simulink model "model_T_PSH_IEEE39"  (R2020b)
settings: Solver=ode3  StartTime=0.0  StopTime=300  FixedStep=Ts  RelTol=1e-3
PostLoadFcn:
  | IEEE39BusLineLength;
  | vNomHV = 345E3;fNom=60;load('Dynamicload.mat');
InitFcn:
  | IEEE39BusLineLength;
  | vNomHV = 345E3;fNom=60;load('Dynamicload.mat');
values from neighbouring files (symbols this model uses):
  At = 1.48    [MAIN_T_PSH_IEEE39.m]
  Dturb = 0.3    [MAIN_T_PSH_IEEE39.m]
  fix_mode = 1    [MAIN_T_PSH_IEEE39.m]
  Gmax = 1    [MAIN_T_PSH_IEEE39.m]
  Gmin = 0    [MAIN_T_PSH_IEEE39.m]
  Hdam = 1    [MAIN_T_PSH_IEEE39.m]
  Kd = 1    [MAIN_T_PSH_IEEE39.m]    (also in plots_T_PSH_IEEE39.m)
  max_delay_gen2pump = 20    [MAIN_T_PSH_IEEE39.m]
  max_delay_pump2hsc = 30    [MAIN_T_PSH_IEEE39.m]
  pgen_pump = Kd*Pref    (= 0.9)    [MAIN_T_PSH_IEEE39.m]
  pgen_turb = (1-Kd)*Pref    (= 0)    [MAIN_T_PSH_IEEE39.m]
  pgen_turb_gen2pump = (1-kd_gen2pump)*Pref    (= 0)    [MAIN_T_PSH_IEEE39.m]
  pgen_turb_hsc2gen = (1-kd_hsc2gen)*Pref    (= 0.36)    [MAIN_T_PSH_IEEE39.m]
  pgen_turb_pump2hsc = (1-kd_pump2hsc)*Pref    (= 0.36)    [MAIN_T_PSH_IEEE39.m]
  Pref = 0.9    [MAIN_T_PSH_IEEE39.m]    (also in MAIN_VS_PSH.m = 1)
  qNL = 0.1    [MAIN_T_PSH_IEEE39.m]
  R = 0.04    [MAIN_T_PSH_IEEE39.m]
  r = 0.31    [MAIN_T_PSH_IEEE39.m]
  Rp = 0.05    [IEEE39BusLineLength.m]
  Sn = 320E6    (= 320000000)    [MAIN_T_PSH_IEEE39.m]
  t_gen2pump = 10    [MAIN_T_PSH_IEEE39.m]
  t_hsc2gen = 150    [MAIN_T_PSH_IEEE39.m]
  t_pump2hsc = 35    [MAIN_T_PSH_IEEE39.m]
  t_sw_off = 220    [MAIN_FS_PSH_IEEE39.m]    (also in MAIN_T_PSH_IEEE39.m; MAIN_VS_PSH.m = 45)
  t_sw_on = 130    [MAIN_FS_PSH_IEEE39.m]    (also in MAIN_T_PSH_IEEE39.m; MAIN_VS_PSH.m = 35)
  Tf = 0.05    [MAIN_T_PSH_IEEE39.m]
  Tg = 0.5    [MAIN_T_PSH_IEEE39.m]
  TL_10_11_len = 14    [IEEE39BusLineLength.m]
  TL_10_13_len = 14    [IEEE39BusLineLength.m]
  TL_13_14_len = 32    [IEEE39BusLineLength.m]
  TL_14_15_len = 70    [IEEE39BusLineLength.m]
  TL_15_16_len = 31.5    [IEEE39BusLineLength.m]
  TL_16_17_len = 26    [IEEE39BusLineLength.m]
  TL_16_19_len = 61    [IEEE39BusLineLength.m]
  TL_16_21_len = 46    [IEEE39BusLineLength.m]
  TL_16_24_len = 15    [IEEE39BusLineLength.m]
  TL_17_18_len = 26    [IEEE39BusLineLength.m]
  TL_17_27_len = 59    [IEEE39BusLineLength.m]
  TL_1_2_len = 134    [IEEE39BusLineLength.m]
  TL_1_39_len = 105    [IEEE39BusLineLength.m]
  TL_21_22_len = 47    [IEEE39BusLineLength.m]
  TL_22_23_len = 33    [IEEE39BusLineLength.m]
  TL_24_23_len = 88    [IEEE39BusLineLength.m]
  TL_25_26_len = 101    [IEEE39BusLineLength.m]
  TL_26_27_len = 46.5    [IEEE39BusLineLength.m]
  TL_26_28_len = 151    [IEEE39BusLineLength.m]
  TL_26_29_len = 200    [IEEE39BusLineLength.m]
  TL_28_29_len = 48    [IEEE39BusLineLength.m]
  TL_2_25_len = 28    [IEEE39BusLineLength.m]
  TL_2_2_len = 49    [IEEE39BusLineLength.m]
  TL_3_18_len = 42    [IEEE39BusLineLength.m]
  TL_3_4_len = 53    [IEEE39BusLineLength.m]
  TL_4_14_len = 33    [IEEE39BusLineLength.m]
  TL_4_5_len = 32.5    [IEEE39BusLineLength.m]
  TL_5_6_len = 14    [IEEE39BusLineLength.m]
  TL_5_8_len = 32    [IEEE39BusLineLength.m]
  TL_6_11_len = 26.5    [IEEE39BusLineLength.m]
  TL_6_7_len = 25.5    [IEEE39BusLineLength.m]
  TL_7_8_len = 15    [IEEE39BusLineLength.m]
  TL_8_9_len = 93    [IEEE39BusLineLength.m]
  TL_9_39_len = 136    [IEEE39BusLineLength.m]
  Tr = 6.88    [MAIN_T_PSH_IEEE39.m]
  Ts = 25e-6    (= 2.5e-05)    [MAIN_FS_PSH_IEEE39.m]    (also in MAIN_T_PSH_IEEE39.m; MAIN_VS_PSH.m = 1e-07)
  Velm = 0.05    [MAIN_T_PSH_IEEE39.m]
  Vn = 18000    [MAIN_T_PSH_IEEE39.m]
undefined symbols (not defined in the file or in its folder): D1, Delta, load15, load16, load18, load20, load21, load23, load24, load25, load26, load27, load28, load29, load3, load39, load4, load7, load8
libraries: powerlib x216, sps_avr x10, simulink_extras x7, powerlib_meascontrol x5, simulink x1
(part 1 of 9)
settings Model: ARTEMISmethode_block_infos=$$__separator__$$IEEE39bus_60Hz/ARTEMIS Guide$$__separator__$$  SimulationMode=accelerator  Creator=Admin  LastModifiedBy=mjimene
settings DataIOCC: LimitDataPoints=on  SaveFormat=Array  SignalLoggingSaveFormat=ModelDataLogs  SaveOutput=off  SignalLogging=off  DSMLogging=off  SaveTime=off
settings OptimizationCC: BlockReduction=off  OptimizeBlockIOStorage=off  BufferReuse=off  GlobalBufferReuse=off  ExpressionFolding=off  ExpressionDepthLimit=2147483647  LocalBlockOutputs=off  LifeSpan=inf
settings DebuggingCC: UnderspecifiedInitializationDetection=Classic  MergeDetectMultiDrivingBlocksExec=none  SolverPrmCheckMsg=warning  FcnCallInpInsideContextMsg=warning  UnconnectedInputMsg=none  UnconnectedOutputMsg=none  UnconnectedLineMsg=none  StateNameClashWarn=warning  SFUnexpectedBacktrackingDiag=warning  SFNoUnconditionalDefaultTransitionDiag=warning  SFExecutionAtInitializationDiag=none  ArithmeticOperatorsInVariantConditions=warning
settings HardwareCC: ProdBitPerPointer=32  ProdBitPerSizeT=32  ProdBitPerPtrDiffT=32  ProdLargestAtomicFloat=None  ProdIntDivRoundTo=Undefined  ProdEndianess=Unspecified  ProdWordSize=32  ProdHWDeviceType=32-bit Generic
settings ModelReferenceCC: PropagateSignalLabelsOutOfModel=off
settings SFSimCC: SimUseLocalCustomCode=off  CustomCodeUndefinedFunction=UseInterfaceOnly
settings RTWCC: RTWUseLocalCustomCode=off
settings CodeAppCC: StateflowObjectComments=on
settings GRTTargetCC: TargetLangStandard=C89/C90 (ANSI)  CombineOutputUpdateFcns=off  GRTInterface=on
settings ConfigComp: CovMetricSettings=dw  CovSaveCumulativeToWorkspaceVar=on  CovSaveSingleToWorkspaceVar=on  CovExternalEMLEnable=off
settings SimscapeCC: SimscapeNormalizeSystem=off

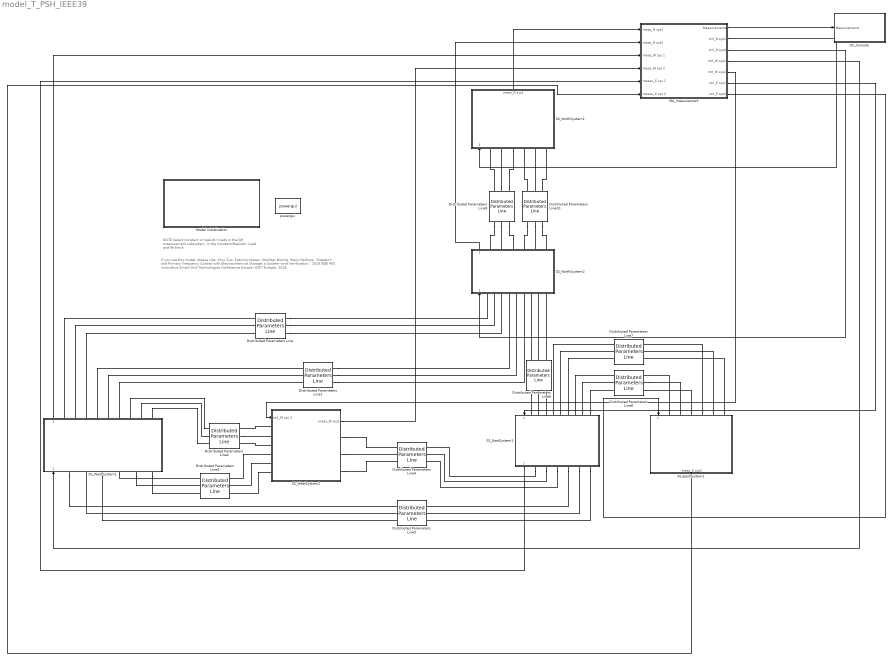
== system model_T_PSH_IEEE39 ==
  note: If you use this model, please cite:
      | Yihui Zuo, Fabrizio Sossan, Mokhtar Bozorg, Mario Paolone,
      | “Dispatch and Primary Frequency Control with Electrochemical Storage: a System-wise Verification,”
      | 2018 IEEE PES Innovative Smart Grid Technologies Conference Europe (ISGT-Europe), 2018.
  note: NOTE
      | Select constant or realistic loads in the SM measurement
      | subsystem, in the Constant/Realistic Load profile block.
  Distributed Parameters Line : powerlib/Elements/Distributed Parameters Line  Phases=3  Length=TL_1_39_len  Frequency=fNom  Resistance=[1.19 4.76]/TL_1_39_len  Inductance="[0.079  0.237]/TL_1_39_len"  Capacitance=[1.67e-6 0.7599e-6]/TL_1_39_len  x1=[-0.000425 6.82447359247909e-09 0 0;-0.0004 6.80872451608349e-09 0 0;-0.000375 6.79237064940765e-09 125916.274403475 -215667.287842067;-0.00035 6.77541344509656e-09 127943.255913456 -214470.993858132;-0.000325 6.75785440938716e-09 129958.872763666 -213255.64932043;-0.0003 6.73969510197452e-09 131962.945915361 -212021.362182889;-0.000275 6.72093713587333e-09 133955.297355178 -210768.242082031;-0.00025 6.7015821772746e-09 135935.75011094 -209496.400327228;-0.000225 6.68163194539767e-09 137904.128267383 -208205.949890819;-0.0002 6.66108821233747e-09 139860.256981778 -206897.005398072;-0.000175 6.63995280290718e-09 141803.962499462 -205569.683117007;-0.00015 6.61822759447605e-09 143735.072169272 -204224.100948063;-0.000125 6.59591451680273e-09 145653.414458882 -202860.378413628;-0.0001 6.57301555186379e-09 147558.818970036 -201478.636647424;-7.5e-05 6.5495327336777e-09 149451.116453689 -200078.998383743;-5e-05 6.52546814812414e-09 151330.138825038 -198661.587946549;-2.5e-05 6.50082393275876e-09 153195.719178451 -197226.531238432]  x2=[-0.000425 -1.36577479152877e-10 0 0;-0.0004 -1.69010241030866e-10 0 0;-0.000375 -2.01427990442011e-10 135245.30623613 -213822.142207347;-0.00035 -2.33827847854369e-10 137254.483681511 -212538.007509997;-0.000325 -2.66206935325264e-10 139251.469390032 -211234.993957904;-0.0003 -2.98562376756929e-10 141236.085977876 -209913.217292266;-0.000275 -3.30891298151972e-10 143208.157159922 -208572.794920929;-0.00025 -3.63190827868667e-10 145167.507765405 -207213.845907958;-0.000225 -3.95458096876025e-10 147113.963753475 -205836.490963062;-0.0002 -4.27690239008639e-10 149047.352228657 -204440.852430872;-0.000175 -4.59884391221277e-10 150967.501456207 -203027.054280071;-0.00015 -4.92037693843189e-10 152874.240877369 -201595.222092386;-0.000125 -5.24147290832123e-10 154767.401124522 -200145.483051432;-0.0001 -5.56210330028012e-10 156646.814036226 -198677.965931411;-7.5e-05 -5.88223963406325e-10 158512.31267216 -197192.80108568;-5e-05 -6.20185347331038e-10 160363.731327948 -195690.120435168;-2.5e-05 -6.52091642807227e-10 162200.90554988 -194170.05745666]  x3=[-0.000425 2.81520374156516e-11 0 0;-0.0004 2.73917536840612e-11 0 0;-0.000375 2.66290368585268e-11 583.079334168895 -1337.51010433723;-0.00035 2.58639546879668e-11 595.658933399881 -1331.95538957714;-0.000325 2.50965751314035e-11 608.185622760243 -1326.28236283785;-0.0003 2.4326966351926e-11 620.658289557001 -1320.49152803039;-0.000275 2.35551967106363e-11 633.075825895772 -1314.58339953019;-0.00025 2.27813347605761e-11 645.437128779179 -1308.5585021314;-0.000225 2.20054492406386e-11 657.741100204826 -1302.41737100023;-0.0002 2.12276090694618e-11 669.986647262827 -1296.16055162746;-0.000175 2.04478833393073e-11 682.172682232888 -1289.78859977996;-0.00015 1.96663413099229e-11 694.298122680923 -1283.30208145135;-0.000125 1.88830524023906e-11 706.361891555199 -1276.70157281168;-0.0001 1.80980861929602e-11 718.362917282012 -1269.98766015629;-7.5e-05 1.73115124068691e-11 730.300133860866 -1263.16093985374;-5e-05 1.65234009121492e-11 742.172480959161 -1256.22201829278;-2.5e-05 1.57338217134204e-11 753.978904006382 -1249.17151182855]  x4=[-0.000425 -1.66454786224224e-11 0 0;-0.0004 -1.59649069897711e-11 0 0;-0.000375 -1.52829172617703e-11 477.711890398408 -711.188785738365;-0.00035 -1.4599570016691e-11 484.393311485576 -706.654944302658;-0.000325 -1.39149259533866e-11 491.031705958008 -702.058333688848;-0.0003 -1.32290458859015e-11 497.626484155121 -697.399362194468;-0.000275 -1.25419907380692e-11 504.177060290586 -692.678443656305;-0.00025 -1.18538215381005e-11 510.682852504353 -687.89599741364;-0.000225 -1.11645994131627e-11 517.143282914341 -683.052448271001;-0.0002 -1.04743855839503e-11 523.557777667766 -678.148226460429;-0.000175 -9.78324135924631e-12 529.925766992116 -673.183767603262;-0.00015 -9.09122813047713e-12 536.246685245757 -668.15951267144;-0.000125 -8.39840736625901e-12 542.519970968182 -663.075907948337;-0.0001 -7.70484060693819e-12 548.745066929881 -657.933404989118;-7.5e-05 -7.01058945912449e-12 554.921420181837 -652.732460580631;-5e-05 -6.31571559021911e-12 561.04848210464 -647.473536700831;-2.5e-05 -5.62028072293689e-12 567.125708457224 -642.157100477745]  x5=0.000424377544174995  V1=ones(3,3)  V2=ones(3,3)  I1=ones(3,3)  I2=ones(3,3)  nHarmo=1  Measurements=None  Decoupling=off  VsMag0=0  VrMag0=0  VsAngle0=0  VrAngle0=0  IsMag0=0  IrMag0=0  IsAngle0=0  IrAngle0=0
  Distributed Parameters Line1 : powerlib/Elements/Distributed Parameters Line  Phases=3  Length=TL_3_4_len  Frequency=fNom  Resistance=[1.547 6.18]/TL_3_4_len  Inductance="[0.067  0.208]/TL_3_4_len"  Capacitance=[0.493e-6 0.224e-6]/TL_3_4_len  x1=[-0.000225 1.6958252968873e-09 0 0;-0.0002 1.54824975012124e-09 116464.900989505 -210886.461836935;-0.000175 1.40053667886024e-09 118447.246041312 -209779.455322648;-0.00015 1.25269920383338e-09 120419.069923853 -208653.814984172;-0.000125 1.10475045682001e-09 122380.197488327 -207509.640807393;-0.0001 9.56703579483276e-10 124330.454536047 -206347.034424475;-7.5e-05 8.08571722202861e-10 126269.667833903 -205166.09910484;-5e-05 6.60368042906836e-10 128197.665129758 -203966.939745992;-2.5e-05 5.12105705902926e-10 130114.275167745 -202749.662864199]  x2=[-0.000225 2.13834554662331e-09 0 0;-0.0002 2.00645197588943e-09 134479.442824576 -206334.576910516;-0.000175 1.87438018048954e-09 136418.087730126 -205057.992053123;-0.00015 1.74214189180416e-09 138344.61519234 -203763.19275921;-0.000125 1.60974885600272e-09 140258.85408591 -202450.294040337;-0.0001 1.47721283300015e-09 142160.634377069 -201119.412515759;-7.5e-05 1.34454559541237e-09 144049.787138696 -199770.666402069;-5e-05 1.21175892751051e-09 145926.14456532 -198404.175502695;-2.5e-05 1.07886462417419e-09 147789.539988023 -197020.06119726]  x3=[-0.000225 -1.78483661113028e-11 0 0;-0.0002 -1.79240452695748e-11 518.089821308726 -1279.69932908716;-0.000175 -1.79981323105074e-11 530.127485951711 -1274.75969133324;-0.00015 -1.80706206532611e-11 542.118061606143 -1269.70682205274;-0.000125 -1.81415038590023e-11 554.060483199762 -1264.54117007074;-0.0001 -1.82107756314747e-11 565.953689937629 -1259.2631942303;-7.5e-05 -1.8278429817559e-11 577.796625396356 -1253.87336335177;-5e-05 -1.83444604078192e-11 589.588237617937 -1248.37215619108;-2.5e-05 -1.84088615370365e-11 601.327479203194 -1242.76006139727]  x4=[-0.000225 2.50482695965397e-11 0 0;-0.0002 2.48471590066135e-11 121.777473885469 128.221815017289;-0.000175 2.46438413483556e-11 120.563589621472 129.363838061733;-0.00015 2.4438334681616e-11 119.338996202334 130.494370262086;-0.000125 2.42306572606851e-11 118.103802403524 131.61331119794;-0.0001 2.40208275326721e-11 116.858117942096 132.720561478492;-7.5e-05 2.38088641358669e-11 115.602053466947 133.81602275137;-5e-05 2.35947858980839e-11 114.335720548986 134.89959771137;-2.5e-05 2.337861183499e-11 113.059231671226 135.971190109098]  x5=0.000215851801011713  V1=ones(3,3)  V2=ones(3,3)  I1=ones(3,3)  I2=ones(3,3)  nHarmo=1  Measurements=None  Decoupling=off  VsMag0=0  VrMag0=0  VsAngle0=0  VrAngle0=0  IsMag0=0  IrMag0=0  IsAngle0=0  IrAngle0=0
  Distributed Parameters Line10 : powerlib/Elements/Distributed Parameters Line  Phases=3  Length=TL_2_25_len  Frequency=fNom  Resistance=[8.33 33.3]/TL_2_25_len  Inductance=[0.027 0.082]/TL_2_25_len  Capacitance=[0.325e-6 0.148e-6]/TL_2_25_len  x1=[-0.000125 -9.05757141638467e-09 0 0;-0.0001 -9.06957005980283e-09 167648.596320969 -188428.534351372;-7.5e-05 -9.08076309156712e-09 169417.00966394 -186840.137060953;-5e-05 -9.09114951744772e-09 171170.374408526 -185235.143549232;-2.5e-05 -9.10072841486225e-09 172908.534810733 -183613.696381013]  x2=[-0.000125 -4.26747363705766e-10 0 0;-0.0001 -6.61699299596901e-10 171332.219594936 -182512.291487725;-7.5e-05 -8.96592459530234e-10 173044.711024908 -180889.440362705;-5e-05 -1.13140597893712e-09 174741.831623084 -179250.521591671;-2.5e-05 -1.36611900032306e-09 176423.4306414 -177595.680752865]  x3=[-0.000125 4.70773669429525e-10 0 0;-0.0001 4.68396340500153e-10 1075.86934502619 -582.792909139489;-7.5e-05 4.65977405899503e-10 1081.31415478568 -572.627345310123;-5e-05 4.63517080491332e-10 1086.66291596967 -562.410917408958;-2.5e-05 4.61015582815971e-10 1091.91515347028 -552.144532918193]  x4=[-0.000125 -4.78403021988109e-10 0 0;-0.0001 -4.7636898850949e-10 52.6144484395538 -697.070225634231;-7.5e-05 -4.74292641182898e-10 59.181687592818 -696.543389127242;-5e-05 -4.72174164441509e-10 65.7436698863957 -695.954681608947;-2.5e-05 -4.70013746460675e-10 72.2998124470777 -695.304155371752]  x5=0.000110163514831363  V1=ones(3,3)  V2=ones(3,3)  I1=ones(3,3)  I2=ones(3,3)  nHarmo=1  Measurements=None  Decoupling=off  VsMag0=0  VrMag0=0  VsAngle0=0  VrAngle0=0  IsMag0=0  IrMag0=0  IsAngle0=0  IrAngle0=0
  Distributed Parameters Line2 : powerlib/Elements/Distributed Parameters Line  Phases=3  Length=TL_5_6_len  Frequency=fNom  Resistance=[0.476 1.904]/TL_5_6_len  Inductance=[0.014 0.04]/TL_5_6_len  Capacitance=[0.162e-6 0.074e-6]/TL_5_6_len  x1=[-7.5e-05 6.48469401785956e-09 0 0;-5e-05 6.33185153631539e-09 132982.125706271 -200175.622617078;-2.5e-05 6.17844662310637e-09 134862.791231139 -198913.421899552]  x2=[-7.5e-05 6.42421610984077e-09 0 0;-5e-05 6.25757145564951e-09 138041.32215589 -196698.021310076;-2.5e-05 6.09037096777966e-09 139888.987836916 -195388.293819903]  x3=[-7.5e-05 1.00931057100308e-10 0 0;-5e-05 1.00601283191749e-10 1184.48127250464 -1575.38524962129;-2.5e-05 1.00262573295529e-10 1199.27604059468 -1564.15196917421]  x4=[-7.5e-05 -8.68602062268655e-11 0 0;-5e-05 -8.69239264867509e-11 -275.774523608809 218.716848838573;-2.5e-05 -8.69799256608829e-11 -277.823617259088 216.10806706858]  x5=5.44058820349418e-05  V1=ones(3,3)  V2=ones(3,3)  I1=ones(3,3)  I2=ones(3,3)  nHarmo=1  Measurements=None  Decoupling=off  VsMag0=0  VrMag0=0  VsAngle0=0  VrAngle0=0  IsMag0=0  IrMag0=0  IsAngle0=0  IrAngle0=0
  Distributed Parameters Line3 : powerlib/Elements/Distributed Parameters Line  Phases=3  Length=TL_7_8_len  Frequency=fNom  Resistance=[0.476 1.904]/TL_7_8_len  Inductance=[0.015 0.044]/TL_7_8_len  Capacitance=[0.174e-6 0.079e-6]/TL_7_8_len  x1=[-7.5e-05 6.07040960241395e-09 122557.52009298 -206550.592006867;-5e-05 5.91980751784004e-09 124498.730220582 -205386.356365422;-2.5e-05 5.76867960173348e-09 126428.881651101 -204203.877120241]  x2=[-7.5e-05 6.76218751498753e-09 124786.001456704 -204826.24564208;-5e-05 6.61873636774516e-09 126710.861311159 -203641.083921901;-2.5e-05 6.47469730606841e-09 128624.465974257 -202437.833623176]  x3=[-7.5e-05 -3.90124045178195e-11 745.609660166508 -1072.1989685999;-5e-05 -3.88230244083392e-11 755.681589498115 -1065.12423419214;-2.5e-05 -3.86301958133523e-11 765.686394821515 -1057.95488929125]  x4=[-7.5e-05 4.65349128222633e-11 82.3065432237965 -335.30367631357;-5e-05 4.58823976117957e-11 85.4629698146192 -334.513076858687;-2.5e-05 4.52258068614755e-11 88.6118050903075 -333.692764018129]  x5=5.89576118919347e-05  V1=ones(3,3)  V2=ones(3,3)  I1=ones(3,3)  I2=ones(3,3)  nHarmo=1  Measurements=None  Decoupling=off  VsMag0=0  VrMag0=0  VsAngle0=0  VrAngle0=0  IsMag0=0  IrMag0=0  IsAngle0=0  IrAngle0=0
  Distributed Parameters Line4 : powerlib/Elements/Distributed Parameters Line  Phases=3  Length=TL_13_14_len  Frequency=fNom  Resistance=[1.071 4.285]/TL_13_14_len  Inductance=[0.032 0.095]/TL_13_14_len  Capacitance=[0.384e-6 0.175e-6]/TL_13_14_len  x1=[-0.00015 -1.84588646488538e-08 0 0;-0.000125 -1.85855470778483e-08 137054.160835711 -198017.584467246;-0.0001 -1.87105786310878e-08 138914.30756397 -196717.103644566;-7.5e-05 -1.88339482025469e-08 140762.115120216 -195399.149271302;-5e-05 -1.89556448338268e-08 142597.419371495 -194063.838415782;-2.5e-05 -1.90756577151292e-08 144420.057295474 -192711.289688038]  x2=[-0.00015 -1.82342608230128e-12 0 0;-0.000125 -1.73806690637535e-10 128270.609996984 -204367.02656213;-0.0001 -3.45774516677539e-10 130190.987834372 -203149.045137268;-7.5e-05 -5.17711629025669e-10 132099.801355444 -201913.018839589;-5e-05 -6.89602755233448e-10 133996.881008345 -200659.057460094;-2.5e-05 -8.61432626937154e-10 135882.058283491 -199387.272382886]  x3=[-0.00015 1.65856168110498e-10 0 0;-0.000125 1.70279111060999e-10 -126.262148596948 -18.9493361137516;-0.0001 1.74686928836284e-10 -126.078020265121 -20.1384817636324;-7.5e-05 1.79079229908492e-10 -125.882692954539 -21.3258385971202;-5e-05 1.83455624128046e-10 -125.676184015303 -22.5113011463157;-2.5e-05 1.87815722758306e-10 -125.458511790729 -23.6947641115808]  x4=[-0.00015 -1.89775651879871e-10 0 0;-0.000125 -1.94616313616103e-10 1013.74461396554 -1390.25070636974;-0.0001 -1.99439688406069e-10 1026.802198003 -1380.63477026534;-7.5e-05 -2.0424534780973e-10 1039.76857553216 -1370.89619819767;-5e-05 -2.09032864960632e-10 1052.6425948044 -1361.03585520302;-2.5e-05 -2.13801814603819e-10 1065.42311227488 -1351.05461713407]  x5=0.000128937969582276  V1=ones(3,3)  V2=ones(3,3)  I1=ones(3,3)  I2=ones(3,3)  nHarmo=1  Measurements=None  Decoupling=off  VsMag0=0  VrMag0=0  VsAngle0=0  VrAngle0=0  IsMag0=0  IrMag0=0  IsAngle0=0  IrAngle0=0
  Distributed Parameters Line5 : powerlib/Elements/Distributed Parameters Line  Phases=3  Length=TL_4_14_len  Frequency=fNom  Resistance=[0.9522 3.808]/TL_4_14_len  Inductance=[0.041 0.1223]/TL_4_14_len  Capacitance=[0.308e-6 0.14e-6]/TL_4_14_len  x1=[-0.00015 1.25269920383338e-09 0 0;-0.000125 1.10475045682001e-09 122380.197488327 -207509.640807393;-0.0001 9.56703579483276e-10 124330.454536047 -206347.034424475;-7.5e-05 8.08571722202861e-10 126269.667833903 -205166.09910484;-5e-05 6.60368042906836e-10 128197.665129758 -203966.939745992;-2.5e-05 5.12105705902926e-10 130114.275167745 -202749.662864199]  x2=[-0.00015 -1.82342608230128e-12 0 0;-0.000125 -1.73806690637535e-10 128270.609996984 -204367.02656213;-0.0001 -3.45774516677539e-10 130190.987834372 -203149.045137268;-7.5e-05 -5.17711629025669e-10 132099.801355444 -201913.018839589;-5e-05 -6.89602755233448e-10 133996.881008345 -200659.057460094;-2.5e-05 -8.61432626937154e-10 135882.058283491 -199387.272382886]  x3=[-0.00015 5.29965279778984e-11 0 0;-0.000125 5.25426459549767e-11 548.434518132287 -941.542402513085;-0.0001 5.20840967904346e-11 557.283853983036 -936.331761920028;-7.5e-05 5.162092121526e-11 566.083688659603 -931.037950925913;-5e-05 5.11531603713857e-11 574.83324050979 -925.661439757641;-2.5e-05 5.06808558080345e-11 583.531732347811 -920.202705988024]  x4=[-0.00015 -5.31610401189671e-11 0 0;-0.000125 -5.30486831737016e-11 113.330971162931 -199.672553983299;-0.0001 -5.29316141376637e-11 115.207723378569 -198.595605403815;-7.5e-05 -5.28098434096022e-11 117.074242178074 -197.50101641436;-5e-05 -5.26833818058973e-11 118.930361766454 -196.388884242657;-2.5e-05 -5.25522405595997e-11 120.775917272435 -195.259307674714]  x5=0.000130851060370178  V1=ones(3,3)  V2=ones(3,3)  I1=ones(3,3)  I2=ones(3,3)  nHarmo=1  Measurements=None  Decoupling=off  VsMag0=0  VrMag0=0  VsAngle0=0  VrAngle0=0  IsMag0=0  IrMag0=0  IsAngle0=0  IrAngle0=0
  Distributed Parameters Line6 : powerlib/Elements/Distributed Parameters Line  Phases=3  Length=TL_16_17_len  Frequency=fNom  Resistance=[0.8332 3.33]/TL_16_17_len  Inductance=[0.028 0.084]/TL_16_17_len  Capacitance=[0.299e-6 0.136e-6]/TL_16_17_len  x1=[-0.000125 3.55201829698564e-08 0 0;-0.0001 3.52355613436191e-08 127482.761229804 -209764.944408129;-7.5e-05 3.49478098910877e-08 129454.048045797 -208554.148041724;-5e-05 3.465695417201e-08 131413.836004727 -207324.826690009;-2.5e-05 3.43630200218728e-08 133361.951026895 -206077.089548415]  x2=[-0.000125 2.39408399520577e-08 0 0;-0.0001 2.36824783705596e-08 131020.122877065 -208712.127601341;-7.5e-05 2.34220131743981e-08 132981.329601984 -207468.039590694;-5e-05 2.31594674995981e-08 134930.724156296 -206205.523069169;-2.5e-05 2.28948646669843e-08 136868.133383506 -204924.690180784]  x3=[-0.000125 -7.51676539007504e-11 0 0;-0.0001 -7.88220241180392e-11 529.194411884565 -1016.0874974886;-7.5e-05 -8.24693929073891e-11 538.747124460212 -1011.05495400868;-5e-05 -8.61094362884146e-11 548.251982401175 -1005.93260278172;-2.5e-05 -8.97418309314155e-11 557.708141431012 -1000.72089880458]  x4=[-0.000125 1.53319636933556e-10 0 0;-0.0001 1.56315144972869e-10 290.26469102285 -363.176651707524;-7.5e-05 1.59296768197176e-10 293.674582186092 -360.424825714346;-5e-05 1.62264241761462e-10 297.058387474888 -357.640984704135;-2.5e-05 1.65217302077566e-10 300.415806320087 -354.825375953746]  x5=0.000106883113727099  V1=ones(3,3)  V2=ones(3,3)  I1=ones(3,3)  I2=ones(3,3)  nHarmo=1  Measurements=None  Decoupling=off  VsMag0=0  VrMag0=0  VsAngle0=0  VrAngle0=0  IsMag0=0  IrMag0=0  IsAngle0=0  IrAngle0=0
  Distributed Parameters Line7 : powerlib/Elements/Distributed Parameters Line  Phases=3  Length=TL_16_21_len  Frequency=fNom  Resistance=[0.9522 3.809]/TL_16_21_len  Inductance=[0.043 0.128]/TL_16_21_len  Capacitance=[0.568e-6 0.258e-6]/TL_16_21_len  x1=[-0.0002 3.63550174769137e-08 0 0;-0.000175 3.60799358967494e-08 121501.663663936 -213285.116380796;-0.00015 3.5801649488061e-08 123506.392436839 -212130.533640322;-0.000125 3.55201829698564e-08 125500.150657839 -210957.10823929;-0.0001 3.52355613436191e-08 127482.761229804 -209764.944408129;-7.5e-05 3.49478098910877e-08 129454.048045797 -208554.148041724;-5e-05 3.465695417201e-08 131413.836004727 -207324.826690009;-2.5e-05 3.43630200218728e-08 133361.951026895 -206077.089548415]  x2=[-0.0002 1.49365973206953e-08 0 0;-0.000175 1.46837342890637e-08 127042.880582269 -205846.70751626;-0.00015 1.44295669632497e-08 128977.258914018 -204640.23140741;-0.000125 1.41741179198648e-08 130900.180739872 -203415.577969956;-0.0001 1.39174098493701e-08 132811.475254794 -202172.855984697;-7.5e-05 1.36594655540607e-08 134710.972686554 -200912.175837386;-5e-05 1.34003079460404e-08 136598.504310808 -199633.649508922;-2.5e-05 1.31399600451864e-08 138473.902466083 -198337.390565408]  x3=[-0.0002 -2.79115737680193e-11 0 0;-0.000175 -3.24004215604224e-11 894.375330557269 -1099.60469305758;-0.00015 -3.68863913600399e-11 904.698963155013 -1091.12669262415;-0.000125 -4.13690846970961e-11 914.942235159789 -1082.55177200889;-0.0001 -4.58481033928492e-11 925.10423670495 -1073.88069288581;-7.5e-05 -5.03230495949607e-11 935.184065142762 -1065.1142254703;-5e-05 -5.47935258128342e-11 945.180825124579 -1056.25314845069;-2.5e-05 -5.92591349529233e-11 955.093628680379 -1047.29824891907]  x4=[-0.0002 1.03978847655996e-10 0 0;-0.000175 1.07755027360876e-10 -38.2016559913804 -446.336261559181;-0.00015 1.11521635641174e-10 -33.993452625192 -446.676471583733;-0.000125 1.15278337924966e-10 -29.7822297639879 -446.977005221351;-0.0001 1.19024800520232e-10 -25.5683614729324 -447.237835776899;-7.5e-05 1.22760690644503e-10 -21.352222052172 -447.4589400819;-5e-05 1.26485676454416e-10 -17.1341860035882 -447.64029849659;-2.5e-05 1.30199427075194e-10 -12.914627997532 -447.781894911666]  x5=0.000181725067065609  V1=ones(3,3)  V2=ones(3,3)  I1=ones(3,3)  I2=ones(3,3)  nHarmo=1  Measurements=None  Decoupling=off  VsMag0=0  VrMag0=0  VsAngle0=0  VrAngle0=0  IsMag0=0  IrMag0=0  IsAngle0=0  IrAngle0=0
  Distributed Parameters Line8 : powerlib/Elements/Distributed Parameters Line  Phases=3  Length=TL_16_24_len  Frequency=fNom  Resistance=[0.357 1.428]/TL_16_24_len  Inductance=[0.019 0.056]/TL_16_24_len  Capacitance=[0.152e-6 0.069e-6]/TL_16_24_len  x1=[-7.5e-05 3.49478098910877e-08 129454.048045797 -208554.148041724;-5e-05 3.465695417201e-08 131413.836004727 -207324.826690009;-2.5e-05 3.43630200218728e-08 133361.951026895 -206077.089548415]  x2=[-7.5e-05 2.9424529652556e-08 129729.694883358 -210501.804918846;-5e-05 2.91892483982628e-08 131707.826547799 -209269.799286697;-2.5e-05 2.89513743861516e-08 133674.259161538 -208019.205100957]  x3=[-7.5e-05 -2.51469137348881e-10 90.694597336161 -645.022035350488;-5e-05 -2.54078013566083e-10 96.7696531139891 -644.138623589418;-2.5e-05 -2.56664321105016e-10 102.836113251696 -643.197995711326]  x4=[-7.5e-05 3.22554721209669e-10 629.831976985986 -546.772388466727;-5e-05 3.24525319269697e-10 634.957095144396 -540.81216044826;-2.5e-05 3.26467091114429e-10 640.025812742229 -534.803894366671]  x5=6.21610810716802e-05  V1=ones(3,3)  V2=ones(3,3)  I1=ones(3,3)  I2=ones(3,3)  nHarmo=1  Measurements=None  Decoupling=off  VsMag0=0  VrMag0=0  VsAngle0=0  VrAngle0=0  IsMag0=0  IrMag0=0  IsAngle0=0  IrAngle0=0
  Distributed Parameters Line9 : powerlib/Elements/Distributed Parameters Line  Phases=3  Length=TL_26_27_len  Frequency=fNom  Resistance=[1.666 6.665]/TL_26_27_len  Inductance=[0.046 0.139]/TL_26_27_len  Capacitance=[0.534e-6 0.243e-6]/TL_26_27_len  x1=[-0.0002 1.52272838880291e-08 0 0;-0.000175 1.49472449786049e-08 127256.586831929 -211796.164829682;-0.00015 1.46658783684552e-08 129247.026043211 -210587.410058936;-0.000125 1.43832090501892e-08 131225.984786321 -209359.949696791;-0.0001 1.40992621321302e-08 133193.287278701 -208113.892773374;-7.5e-05 1.38140628360853e-08 135148.758773167 -206849.349970666;-5e-05 1.3527636495105e-08 137092.225573436 -205566.433612669;-2.5e-05 1.3240008551233e-08 139023.515049548 -204265.257655433]  x2=[-0.0002 9.02877067542436e-09 0 0;-0.000175 8.71213522248572e-09 141750.530907737 -204239.085171132;-0.00015 8.39472590732218e-09 143669.103226295 -202894.065812053;-0.000125 8.07657092406441e-09 145574.914024395 -201531.024228895;-0.0001 7.75769853307762e-09 147467.794016903 -200150.081494893;-7.5e-05 7.43813705845132e-09 149347.575067272 -198751.360273364;-5e-05 7.11791488548344e-09 151214.090202481 -197334.984806816;-2.5e-05 6.79706045815894e-09 153067.173627864 -195901.080905906]  x3=[-0.0002 8.02462137756003e-11 0 0;-0.000175 7.87138233867969e-11 920.624462147512 -1516.26187198719;-0.00015 7.71744411810691e-11 934.873751756558 -1507.51799994247;-0.000125 7.56282038952452e-11 949.040000473439 -1498.64022143237;-0.0001 7.40752488750614e-11 963.121949970034 -1489.62932503252;-7.5e-05 7.25157140629621e-11 977.118349406165 -1480.48611114283;-5e-05 7.09497379858465e-11 991.027955540705 -1471.21139191643;-2.5e-05 6.93774597427646e-11 1004.84953284201 -1461.80599118751]  x4=[-0.0002 -4.44685173545744e-11 0 0;-0.000175 -4.36928200540542e-11 -49.7397106711078 77.7795104983289;-0.00015 -4.29132417046206e-11 -50.4705805078938 77.3073039358754;-0.000125 -4.21298515529301e-11 -51.1969672558932 76.8282304916876;-0.0001 -4.13427191842256e-11 -51.9188063932348 76.342332719839;-7.5e-05 -4.05519145161555e-11 -52.6360338019929 75.8496537805793;-5e-05 -3.97575077925628e-11 -53.3485857738819 75.3502374365004;-2.5e-05 -3.8959569577246e-11 -54.0563990159155 74.8441280486498]  x5=0.000183785200709959  V1=ones(3,3)  V2=ones(3,3)  I1=ones(3,3)  I2=ones(3,3)  nHarmo=1  Measurements=None  Decoupling=off  VsMag0=0  VrMag0=0  VsAngle0=0  VrAngle0=0  IsMag0=0  IrMag0=0  IsAngle0=0  IrAngle0=0
  Model Initialization : Subsystem  AncestorBlock=artemis/Tools /Misc/Model Initialization  mask(Model Functions){InitFcnX=|, prel=off, posl=on, inif=on, strf=off}
      mask InitFcnX=|
      | IEEE39BusLineLength;
      | vNomHV = 345E3;fNom=60;load('Dynamicload.mat');
      mask prompts: InitFcnX "Initialisation"; prel "Preload Function"; posl "PostLoad Function"; inif "InitFcn"; strf "StartFcn"
      mask init:
      | currentBlock = gcb;
      | root = bdroot(currentBlock);
      | 
      | if ~strcmp(get_param(root,'BlockDiagramType'),'library')
      |     if prel==1
      |         set_param(root, 'PreLoadFcn', InitFcnX);
      |     else
      |         set_param(root, 'PreLoadFcn', '');
      |     end
      |     if inif==1
      |         set_param(root, 'InitFcn', InitFcnX);
      |     else
      |         set_param(root, 'InitFcn', '');
      |     end
      |     if strf==1
      |         set_param(root, 'StartFcn', InitFcnX);
      |     else
      |         set_param(root, 'StartFcn', '');
      |     end
      |     if posl==1
      |         set_param(root, 'PostLoadFcn', InitFcnX);
      |     else
      |         set_param(root, 'PostLoadFcn', '');
      |     end
      | end
      | 
      | pos = get_param(currentBlock, 'Position');
      | width = pos(3) - pos(1); height = pos(4) - pos(2);
      | txt = [ upper(root) '\n' '- InitFcn. . . . . '  get_param(root, 'InitFcn') ];
      settings: CopyFcn=set_param(gcb,'LinkStatus','inactive')
      mask Display: text(5, height*0.5, txt, 'horizontalAlignment', 'left', 'verticalAlignment', 'middle') ;
  SC_Console : Subsystem
  SM_measurement : Subsystem
  SS_EastSystem1 : Subsystem
      mask Display: disp('Eastsystem 1')
  SS_EastSystem2 : Subsystem
      mask Display: disp('Eastsystem 2')
  SS_NorthSystem1 : Subsystem
      mask Display: disp('Northsystem 1')
  SS_NorthSystem2 : Subsystem
      mask Display: disp('Northsystem 2')
  SS_WestSystem1 : Subsystem
      mask Display: disp('WestSystem 1')
  SS_WestSystem2 : Subsystem
      mask Display: disp('Westsystem 2')
  powergui : powerlib/powergui  SimulationMode=Discrete  SampleTime=Ts  frequency=60  Iterations=50  frequencyindice=0  Pbase=100e6  ErrMax=0.0001  UnitsV=kV  UnitsW=MW  buscounter=0  FunctionMessages=off  echomessages=off  EnableUseOfTLC=off  CurrentSourceSwitches=off  DisableSnubberDevices=off  DisableRonSwitches=off  DisableVfSwitches=off  DisplayEquations=off  AutomaticDiscreteSolvers=off  SolverType=Tustin  Interpol=off  ExternalGateDelay=off  methode=off  Ts=0  x0status=steady  SPID=off  SwTol=0  HookPort=off  NonlinearTolerance=1e-4  nMaxIteration=100  ContinueOnMaxIteration=off  RestoreLinks=warning  ResistiveCurrentMeasurement=off  Frange=[0:2:500]  Ylog=off  Xlog=on  ShowGrid=off  save=off  variable=ZData  structure=0  ZoomFFT=on  StartTime=0.0  cycles=1  DisplayStyle=1  fundamental=60  FreqAxis=off  MaxFrequency=1000  frequencyindicesteady=1  RmsSteady=2  display=off
  wires:
  SM_measurement/1(Measurements) -> SC_Console/1(Measurements)
  SM_measurement/5(ctrl_W sys2) -> SS_WestSystem2/1(ctrl_W sys 2)
  SM_measurement/6(ctrl_E sys1) -> SS_EastSystem1/1(ctrl_E sys1)
  SM_measurement/4(ctrl_W sys1) -> SS_WestSystem1/1(ctrl_W sys 1)
  SS_NorthSystem1/1(meas_N sys1) -> SM_measurement/1(meas_N sys1)
  SS_NorthSystem2/1(meas_N sys2) -> SM_measurement/2(" meas_N sys2")
  SS_EastSystem2/1(meas_E sys2) -> SM_measurement/6(measu_E sys 2)
  SS_EastSystem1/1(meas_E sys1) -> SM_measurement/5(measu_E sys 1)
  SS_WestSystem1/1(meas_W sys1) -> SM_measurement/3("meas_W sys 1  ")
  SS_WestSystem2/1(meas_W sys2) -> SM_measurement/4(" meas_W sys 2  ")
  SM_measurement/7(ctrl_E sys2) -> SS_EastSystem2/1(ctrl_E sys2)
  SM_measurement/3(ctrl_N sys2) -> SS_NorthSystem2/1(ctrl_N sys2)
  SM_measurement/2(ctrl_N sys1) -> SS_NorthSystem1/1(ctrl_N sys1)
  connections:
  Distributed Parameters Line/LConn1 -- SS_WestSystem1/RConn1
  Distributed Parameters Line/LConn2 -- SS_WestSystem1/RConn2
  Distributed Parameters Line/LConn3 -- SS_WestSystem1/RConn3
  Distributed Parameters Line1/LConn1 -- SS_WestSystem1/RConn4
  Distributed Parameters Line1/LConn2 -- SS_WestSystem1/RConn5
  Distributed Parameters Line1/LConn3 -- SS_WestSystem1/RConn6
  Distributed Parameters Line6/LConn2 -- SS_EastSystem1/LConn2
  Distributed Parameters Line6/LConn1 -- SS_EastSystem1/LConn1
  Distributed Parameters Line6/LConn3 -- SS_EastSystem1/LConn3
  SS_EastSystem1/RConn1 -- Distributed Parameters Line4/RConn1
  SS_EastSystem1/RConn2 -- Distributed Parameters Line4/RConn2
  SS_EastSystem1/RConn3 -- Distributed Parameters Line4/RConn3
  SS_EastSystem1/RConn4 -- Distributed Parameters Line5/RConn1
  SS_EastSystem1/RConn5 -- Distributed Parameters Line5/RConn2
  SS_EastSystem1/RConn6 -- Distributed Parameters Line5/RConn3
  Distributed Parameters Line/RConn1 -- SS_NorthSystem2/LConn1
  Distributed Parameters Line/RConn2 -- SS_NorthSystem2/LConn2
  Distributed Parameters Line/RConn3 -- SS_NorthSystem2/LConn3
  Distributed Parameters Line1/RConn1 -- SS_NorthSystem2/LConn4
  Distributed Parameters Line1/RConn2 -- SS_NorthSystem2/LConn5
  Distributed Parameters Line1/RConn3 -- SS_NorthSystem2/LConn6
  SS_WestSystem1/LConn1 -- Distributed Parameters Line5/LConn1
  Distributed Parameters Line5/LConn2 -- SS_WestSystem1/LConn2
  SS_WestSystem1/LConn3 -- Distributed Parameters Line5/LConn3
  Distributed Parameters Line6/RConn1 -- SS_NorthSystem2/LConn7
  Distributed Parameters Line6/RConn2 -- SS_NorthSystem2/LConn8
  Distributed Parameters Line6/RConn3 -- SS_NorthSystem2/LConn9
  Distributed Parameters Line9/RConn2 -- SS_NorthSystem1/LConn2
  Distributed Parameters Line9/LConn2 -- SS_NorthSystem2/RConn2
  Distributed Parameters Line10/RConn2 -- SS_NorthSystem1/LConn5
  Distributed Parameters Line10/LConn2 -- SS_NorthSystem2/RConn5
  Distributed Parameters Line10/RConn3 -- SS_NorthSystem1/LConn6
  Distributed Parameters Line10/RConn1 -- SS_NorthSystem1/LConn4
  Distributed Parameters Line9/RConn3 -- SS_NorthSystem1/LConn3
  Distributed Parameters Line9/RConn1 -- SS_NorthSystem1/LConn1
  Distributed Parameters Line9/LConn1 -- SS_NorthSystem2/RConn1
  Distributed Parameters Line9/LConn3 -- SS_NorthSystem2/RConn3
  SS_EastSystem1/LConn7 -- Distributed Parameters Line8/LConn1
  Distributed Parameters Line8/LConn2 -- SS_EastSystem1/LConn8
  SS_EastSystem1/LConn9 -- Distributed Parameters Line8/LConn3
  SS_EastSystem2/LConn3 -- Distributed Parameters Line8/RConn3
  Distributed Parameters Line8/RConn2 -- SS_EastSystem2/LConn2
  SS_EastSystem2/LConn1 -- Distributed Parameters Line8/RConn1
  SS_EastSystem1/LConn4 -- Distributed Parameters Line7/LConn1
  SS_EastSystem1/LConn5 -- Distributed Parameters Line7/LConn2
  SS_EastSystem1/LConn6 -- Distributed Parameters Line7/LConn3
  SS_EastSystem2/LConn4 -- Distributed Parameters Line7/RConn1
  SS_EastSystem2/LConn5 -- Distributed Parameters Line7/RConn2
  SS_EastSystem2/LConn6 -- Distributed Parameters Line7/RConn3
  SS_WestSystem2/RConn1 -- Distributed Parameters Line4/LConn1
  SS_WestSystem2/RConn2 -- Distributed Parameters Line4/LConn2
  SS_WestSystem2/RConn3 -- Distributed Parameters Line4/LConn3
  SS_WestSystem1/RConn7 -- Distributed Parameters Line2/LConn1
  Distributed Parameters Line2/LConn2 -- SS_WestSystem1/RConn8
  SS_WestSystem1/RConn9 -- Distributed Parameters Line2/LConn3
  SS_WestSystem2/LConn1 -- Distributed Parameters Line2/RConn1
  Distributed Parameters Line2/RConn2 -- SS_WestSystem2/LConn2
  SS_WestSystem2/LConn3 -- Distributed Parameters Line2/RConn3
  SS_WestSystem2/LConn4 -- Distributed Parameters Line3/RConn1
  SS_WestSystem2/LConn5 -- Distributed Parameters Line3/RConn2
  SS_WestSystem2/LConn6 -- Distributed Parameters Line3/RConn3
  Distributed Parameters Line3/LConn1 -- SS_WestSystem1/LConn4
  SS_WestSystem1/LConn5 -- Distributed Parameters Line3/LConn2
  SS_WestSystem1/LConn6 -- Distributed Parameters Line3/LConn3
  Distributed Parameters Line10/LConn1 -- SS_NorthSystem2/RConn4
  Distributed Parameters Line10/LConn3 -- SS_NorthSystem2/RConn6

== system model_T_PSH_IEEE39/Model Initialization ==

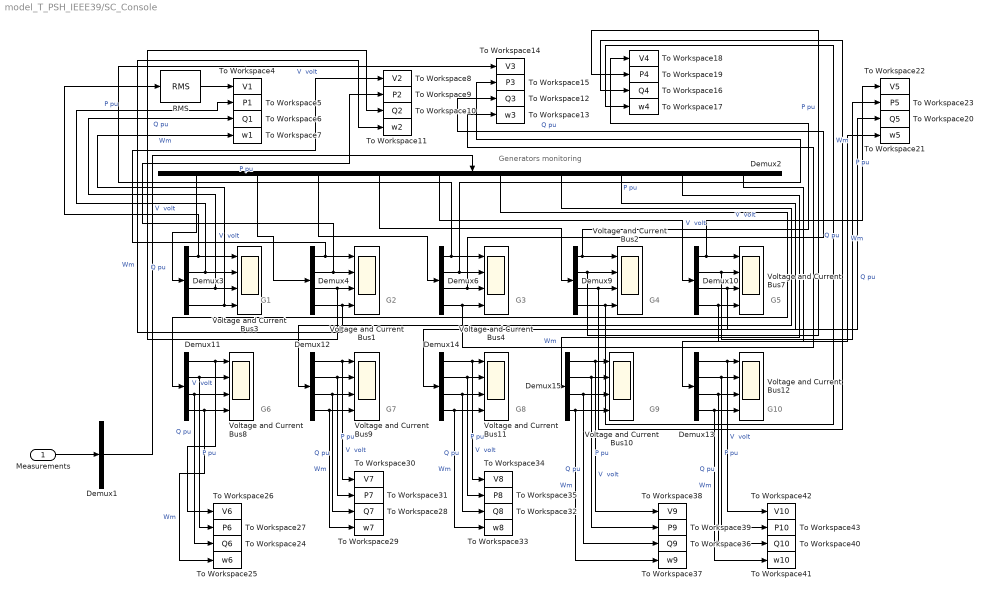
== system model_T_PSH_IEEE39/SC_Console ==
  note: G10
  note: G9
  note: G8
  note: G7
  note: G6
  note: G5
  note: G4
  note: G3
  note: G2
  note: G1
  note: Generators monitoring
  Measurements : Inport
  Demux1 : Demux  Outputs=[60 ]
  Demux{3..4,6,9..15} (10 alike) : Demux  Outputs=[3 1 1 1]
  Demux2 : Demux  Outputs=[6 6 6 6 6 6 6 6 6 6]
  RMS : powerlib_meascontrol/Measurements/RMS  TrueRMS=on  Freq=60  RMSInit=120  Ts=0
  To Workspace10 : ToWorkspace  VariableName=Q2  SaveFormat=Timeseries  SampleTime=-1
  To Workspace11 : ToWorkspace  VariableName=w2  SaveFormat=Timeseries  SampleTime=-1
  To Workspace12 : ToWorkspace  VariableName=Q3  SaveFormat=Timeseries  SampleTime=-1
  To Workspace13 : ToWorkspace  VariableName=w3  SaveFormat=Timeseries  SampleTime=-1
  To Workspace14 : ToWorkspace  VariableName=V3  SaveFormat=Timeseries  SampleTime=-1
  To Workspace15 : ToWorkspace  VariableName=P3  SaveFormat=Timeseries  SampleTime=-1
  To Workspace16 : ToWorkspace  VariableName=Q4  SaveFormat=Timeseries  SampleTime=-1
  To Workspace17 : ToWorkspace  VariableName=w4  SaveFormat=Timeseries  SampleTime=-1
  To Workspace18 : ToWorkspace  VariableName=V4  SaveFormat=Timeseries  SampleTime=-1
  To Workspace19 : ToWorkspace  VariableName=P4  SaveFormat=Timeseries  SampleTime=-1
  To Workspace20 : ToWorkspace  VariableName=Q5  SaveFormat=Timeseries  SampleTime=-1
  To Workspace21 : ToWorkspace  VariableName=w5  SaveFormat=Timeseries  SampleTime=-1
  To Workspace22 : ToWorkspace  VariableName=V5  SaveFormat=Timeseries  SampleTime=-1
  To Workspace23 : ToWorkspace  VariableName=P5  SaveFormat=Timeseries  SampleTime=-1
  To Workspace24 : ToWorkspace  VariableName=Q6  SaveFormat=Timeseries  SampleTime=-1
  To Workspace25 : ToWorkspace  VariableName=w6  SaveFormat=Timeseries  SampleTime=-1
  To Workspace26 : ToWorkspace  VariableName=V6  SaveFormat=Timeseries  SampleTime=-1
  To Workspace27 : ToWorkspace  VariableName=P6  SaveFormat=Timeseries  SampleTime=-1
  To Workspace28 : ToWorkspace  VariableName=Q7  SaveFormat=Timeseries  SampleTime=-1
  To Workspace29 : ToWorkspace  VariableName=w7  SaveFormat=Timeseries  SampleTime=-1
  To Workspace30 : ToWorkspace  VariableName=V7  SaveFormat=Timeseries  SampleTime=-1
  To Workspace31 : ToWorkspace  VariableName=P7  SaveFormat=Timeseries  SampleTime=-1
  To Workspace32 : ToWorkspace  VariableName=Q8  SaveFormat=Timeseries  SampleTime=-1
  To Workspace33 : ToWorkspace  VariableName=w8  SaveFormat=Timeseries  SampleTime=-1
  To Workspace34 : ToWorkspace  VariableName=V8  SaveFormat=Timeseries  SampleTime=-1
  To Workspace35 : ToWorkspace  VariableName=P8  SaveFormat=Timeseries  SampleTime=-1
  To Workspace36 : ToWorkspace  VariableName=Q9  SaveFormat=Timeseries  SampleTime=-1
  To Workspace37 : ToWorkspace  VariableName=w9  SaveFormat=Timeseries  SampleTime=-1
  To Workspace38 : ToWorkspace  VariableName=V9  SaveFormat=Timeseries  SampleTime=-1
  To Workspace39 : ToWorkspace  VariableName=P9  SaveFormat=Timeseries  SampleTime=-1
  To Workspace4 : ToWorkspace  VariableName=V1  SaveFormat=Timeseries  SampleTime=-1
  To Workspace40 : ToWorkspace  VariableName=Q10  SaveFormat=Timeseries  SampleTime=-1
  To Workspace41 : ToWorkspace  VariableName=w10  SaveFormat=Timeseries  SampleTime=-1
  To Workspace42 : ToWorkspace  VariableName=V10  SaveFormat=Timeseries  SampleTime=-1
  To Workspace43 : ToWorkspace  VariableName=P10  SaveFormat=Timeseries  SampleTime=-1
  To Workspace5 : ToWorkspace  VariableName=P1  SaveFormat=Timeseries  SampleTime=-1
  To Workspace6 : ToWorkspace  VariableName=Q1  SaveFormat=Timeseries  SampleTime=-1
  To Workspace7 : ToWorkspace  VariableName=w1  SaveFormat=Timeseries  SampleTime=-1
  To Workspace8 : ToWorkspace  VariableName=V2  SaveFormat=Timeseries  SampleTime=-1
  To Workspace9 : ToWorkspace  VariableName=P2  SaveFormat=Timeseries  SampleTime=-1
  Voltage and Current Bus{1..4,7..12} (10 alike) : Scope  NumInputPorts=4
  wires:
  Demux1/1 -> Demux2/1
  Demux2/10 -> Demux13/1
  Demux2/9 -> Demux15/1
  Demux2/8 -> Demux14/1
  Demux2/7 -> Demux12/1
  Demux2/6 -> Demux11/1
  Demux2/5 -> Demux10/1
  Demux2/4 -> Demux9/1
  Demux2/3 -> Demux6/1
  Demux2/2 -> Demux4/1
  Demux2/1 -> Demux3/1
  Measurements/1 -> Demux1/1
  Demux3/1 -> Voltage and Current Bus3/1, RMS/1  "V  volt"
  Demux3/3 -> To Workspace6/1, Voltage and Current Bus3/3  "Q pu"
  Demux3/4 -> To Workspace7/1, Voltage and Current Bus3/4  "Wm"
  Demux3/2 -> To Workspace5/1, Voltage and Current Bus3/2  "P pu"
  Demux4/1 -> To Workspace8/1, Voltage and Current Bus1/1  "V  volt"
  Demux4/3 -> To Workspace10/1, Voltage and Current Bus1/3  "Q pu"
  Demux4/4 -> To Workspace11/1, Voltage and Current Bus1/4  "Wm"
  Demux4/2 -> To Workspace9/1, Voltage and Current Bus1/2  "P pu"
  Demux6/1 -> To Workspace14/1, Voltage and Current Bus4/1  "V  volt"
  Demux6/3 -> To Workspace12/1, Voltage and Current Bus4/3  "Q pu"
  Demux6/4 -> To Workspace13/1, Voltage and Current Bus4/4  "Wm"
  Demux6/2 -> To Workspace15/1, Voltage and Current Bus4/2  "P pu"
  Demux9/1 -> To Workspace18/1, Voltage and Current Bus2/1  "V  volt"
  Demux9/3 -> To Workspace16/1, Voltage and Current Bus2/3  "Q pu"
  Demux9/4 -> To Workspace17/1, Voltage and Current Bus2/4  "Wm"
  Demux9/2 -> To Workspace19/1, Voltage and Current Bus2/2  "P pu"
  Demux10/1 -> To Workspace22/1, Voltage and Current Bus7/1  "V  volt"
  Demux10/3 -> To Workspace20/1, Voltage and Current Bus7/3  "Q pu"
  Demux10/4 -> To Workspace21/1, Voltage and Current Bus7/4  "Wm"
  Demux10/2 -> To Workspace23/1, Voltage and Current Bus7/2  "P pu"
  Demux11/1 -> To Workspace26/1, Voltage and Current Bus8/1  "V  volt"
  Demux11/3 -> Voltage and Current Bus8/3, To Workspace24/1  "Q pu"
  Demux11/4 -> To Workspace25/1, Voltage and Current Bus8/4  "Wm"
  Demux11/2 -> Voltage and Current Bus8/2, To Workspace27/1  "P pu"
  Demux12/1 -> To Workspace30/1, Voltage and Current Bus9/1  "V  volt"
  Demux12/3 -> To Workspace28/1, Voltage and Current Bus9/3  "Q pu"
  Demux12/4 -> To Workspace29/1, Voltage and Current Bus9/4  "Wm"
  Demux12/2 -> To Workspace31/1, Voltage and Current Bus9/2  "P pu"
  Demux14/1 -> To Workspace34/1, Voltage and Current Bus11/1  "V  volt"
  Demux14/3 -> To Workspace32/1, Voltage and Current Bus11/3  "Q pu"
  Demux14/4 -> To Workspace33/1, Voltage and Current Bus11/4  "Wm"
  Demux14/2 -> To Workspace35/1, Voltage and Current Bus11/2  "P pu"
  Demux15/1 -> To Workspace38/1, Voltage and Current Bus10/1  "V  volt"
  Demux15/3 -> To Workspace36/1, Voltage and Current Bus10/3  "Q pu"
  Demux15/4 -> To Workspace37/1, Voltage and Current Bus10/4  "Wm"
  Demux15/2 -> To Workspace39/1, Voltage and Current Bus10/2  "P pu"
  Demux13/1 -> To Workspace42/1, Voltage and Current Bus12/1  "V  volt"
  Demux13/3 -> To Workspace40/1, Voltage and Current Bus12/3  "Q pu"
  Demux13/4 -> To Workspace41/1, Voltage and Current Bus12/4  "Wm"
  Demux13/2 -> To Workspace43/1, Voltage and Current Bus12/2  "P pu"
  RMS/1 -> To Workspace4/1

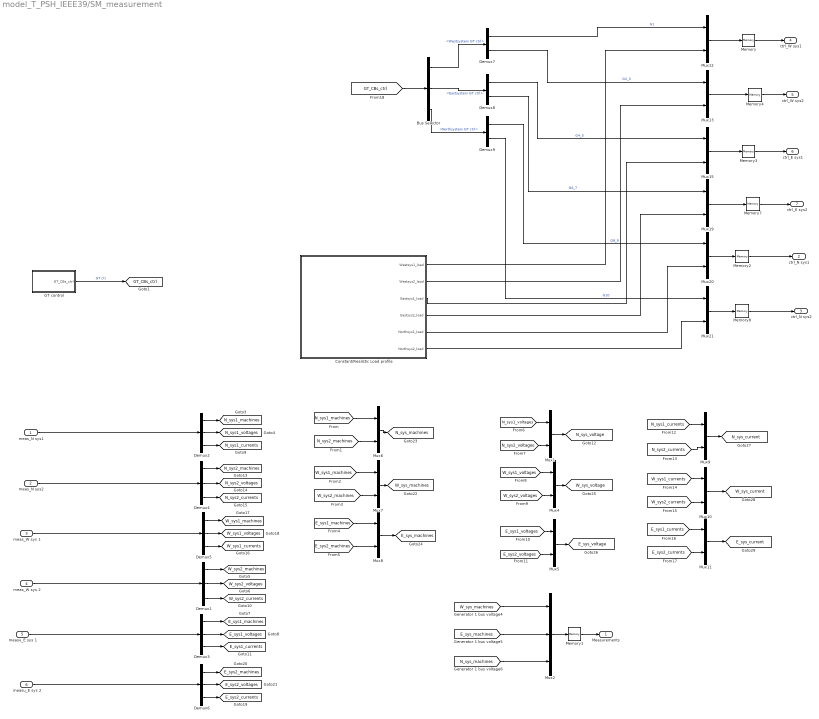
== system model_T_PSH_IEEE39/SM_measurement ==
  meas_N sys1 : Inport
  " meas_N sys2" : Inport  Port=2
  "meas_W sys 1  " : Inport  Port=3
  " meas_W sys 2  " : Inport  Port=4
  measu_E sys 1 : Inport  Port=5
  measu_E sys 2 : Inport  Port=6
  Bus Selector : BusSelector  OutputSignals=Westsystem GT ctrl,Eastsystem GT ctrl,Northsystem GT ctrl
  Constant/Realistic Load profile : Subsystem  SystemSampleTime=20e-3  mask{Loadselect=Constant Load}
      mask init:
      | if (Loadselect == 1)
      |     mode = 0;
      | else 
      |         mode = 1; 
      | end
      mask TypeOptions Loadselect: Constant Load | Realistic Load
      mask Display: disp('Load Profile \n Constant / Realistic')
  Demux1 : Demux  Outputs=[12 18 18]
  Demux2 : Demux  Outputs=[12 12 12]
  Demux3 : Demux  Outputs=[12 15 15]
  Demux4 : Demux  Outputs=[6 18 18]
  Demux5 : Demux  Outputs=[6 15 15]
  Demux6 : Demux  Outputs=[12 12 12]
  Demux7 : Demux  Outputs=[1 2]
  Demux8 : Demux  Outputs=[2 2]
  Demux9 : Demux  Outputs=[2 1]
  GT control : Subsystem
  Memory{,1..4,7..8} (7 alike) : Memory
  Mux{1,4..13,15,19..21} (15 alike) : Mux  Inputs=2
  Mux2 : Mux  Inputs=3
  Measurements : Outport
  ctrl_N sys1 : Outport  Port=2
  ctrl_N sys2 : Outport  Port=3
  ctrl_W sys1 : Outport  Port=4
  ctrl_W sys2 : Outport  Port=5
  ctrl_E sys1 : Outport  Port=6
  ctrl_E sys2 : Outport  Port=7
  tag scope: E_sys1_currents=global, E_sys1_machines=global, E_sys1_voltages=global, E_sys2_currents=global, E_sys2_machines=global, E_sys2_voltages=global, E_sys_current=global, E_sys_machines=global, E_sys_voltage=global, GT_CBs_ctrl=global, N_sys1_currents=global, N_sys1_machines=global, N_sys1_voltages=global, N_sys2_currents=global, N_sys2_machines=global, N_sys2_voltages=global, N_sys_current=global, N_sys_machines=global, N_sys_voltage=global, W_sys1_currents=global, W_sys1_machines=global, W_sys1_voltages=global, W_sys2_currents=global, W_sys2_machines=global, W_sys2_voltages=global, W_sys_current=global, W_sys_machines=global, W_sys_voltage=global
  wires:
  Demux3/2 -> [E_sys1_voltages]
  Demux1/2 -> [W_sys2_voltages]
  Demux2/2 -> [N_sys1_voltages]
  Memory1/1 -> Measurements/1
  [N_sys_machines] -> Mux2/3
  [E_sys_machines] -> Mux2/2
  [W_sys_machines] -> Mux2/1
  Demux3/1 -> [E_sys1_machines]
  Demux1/1 -> [W_sys2_machines]
  Mux2/1 -> Memory1/1
  meas_N sys1/1 -> Demux2/1
  Demux2/1 -> [N_sys1_machines]
  Demux2/3 -> [N_sys1_currents]
  Demux1/3 -> [W_sys2_currents]
  Demux3/3 -> [E_sys1_currents]
  GT control/1(GT_CBs_ctrl) -> [GT_CBs_ctrl]  "GT ctr"
  Demux4/2 -> [N_sys2_voltages]
  Demux4/1 -> [N_sys2_machines]
  Demux4/3 -> [N_sys2_currents]
  " meas_N sys2"/1 -> Demux4/1
  " meas_W sys 2  "/1 -> Demux1/1
  Demux5/2 -> [W_sys1_voltages]
  Demux5/1 -> [W_sys1_machines]
  Demux5/3 -> [W_sys1_currents]
  "meas_W sys 1  "/1 -> Demux5/1
  measu_E sys 1/1 -> Demux3/1
  Demux6/2 -> [E_sys2_voltages]
  Demux6/1 -> [E_sys2_machines]
  Demux6/3 -> [E_sys2_currents]
  measu_E sys 2/1 -> Demux6/1
  [N_sys2_machines] -> Mux6/2
  [N_sys1_machines] -> Mux6/1
  Mux6/1 -> [N_sys_machines]
  [W_sys1_machines] -> Mux7/1
  [W_sys2_machines] -> Mux7/2
  Mux7/1 -> [W_sys_machines]
  [E_sys1_machines] -> Mux8/1
  [E_sys2_machines] -> Mux8/2
  Mux8/1 -> [E_sys_machines]
  [N_sys1_voltages] -> Mux1/1
  [N_sys2_voltages] -> Mux1/2
  [W_sys1_voltages] -> Mux4/1
  [W_sys2_voltages] -> Mux4/2
  [E_sys1_voltages] -> Mux5/1
  [E_sys2_voltages] -> Mux5/2
  Mux1/1 -> [N_sys_voltage]
  Mux4/1 -> [W_sys_voltage]
  Mux5/1 -> [E_sys_voltage]
  [N_sys1_currents] -> Mux9/1
  [N_sys2_currents] -> Mux9/2
  [W_sys1_currents] -> Mux10/1
  [W_sys2_currents] -> Mux10/2
  [E_sys1_currents] -> Mux11/1
  [E_sys2_currents] -> Mux11/2
  Mux9/1 -> [N_sys_current]
  Mux10/1 -> [W_sys_current]
  Mux11/1 -> [E_sys_current]
  Memory2/1 -> ctrl_N sys1/1
  Memory3/1 -> ctrl_E sys1/1
  Memory/1 -> ctrl_W sys1/1
  Constant/Realistic Load profile/1(Westsys1_load) -> Mux12/2
  Constant/Realistic Load profile/2(Westsys2_laod) -> Mux13/2
  Memory4/1 -> ctrl_W sys2/1
  Constant/Realistic Load profile/3(Eastsys1_load) -> Mux15/2
  Constant/Realistic Load profile/4(Eastsys2_load) -> Mux19/2
  Memory7/1 -> ctrl_E sys2/1
  Constant/Realistic Load profile/5(Northsys1_load) -> Mux20/2
  Constant/Realistic Load profile/6(Northsys2_load) -> Mux21/2
  Memory8/1 -> ctrl_N sys2/1
  Mux20/1 -> Memory2/1
  [GT_CBs_ctrl] -> Bus Selector/1
  Bus Selector/2 -> Demux8/1  "<Eastsystem GT ctrl>"
  Bus Selector/1 -> Demux7/1  "<Westsystem GT ctrl>"
  Bus Selector/3 -> Demux9/1  "<Northsystem GT ctrl>"
  Demux7/1 -> Mux12/1  "G1"
  Mux12/1 -> Memory/1
  Demux7/2 -> Mux13/1  "G2_3"
  Mux13/1 -> Memory4/1
  Demux8/1 -> Mux15/1  "G4_5"
  Demux8/2 -> Mux19/1  "G6_7"
  Mux15/1 -> Memory3/1
  Mux19/1 -> Memory7/1
  Demux9/1 -> Mux20/1  "G8_9"
  Demux9/2 -> Mux21/1  "G10"
  Mux21/1 -> Memory8/1
